simulink model "cruise_control_fechada"  (R2021b)
settings: Solver=FixedStepAuto  StartTime=0.0  StopTime=100.0  FixedStep=1e-3  RelTol=1e-3
values from neighbouring files (symbols this model uses):
  b = b_car + delta_b    [closedDrag.m]    (also in identificarCruiseControl.m = f/v_inf; openDrag.m)
  bc = b    [closedDistur.m]    (also in closedDrag.m = b_car; closedFf.m = 0; closedU.m; closedVelRef.m)
  d = 300    [closedDistur.m]    (also in closedDrag.m = 0; closedFf.m = 0; closedU.m = 0; closedVelRef.m = 0)
  Kp = m/tau - b    [closedDistur.m]    (also in closedDrag.m = m/tau - b_car; closedFf.m; closedU.m; closedVelRef.m)
  m = tau*b    [identificarCruiseControl.m]    (also in openMass.m = m_car + m_pass)
  vr = 10    [closedDistur.m]    (also in closedDrag.m; closedFf.m; closedU.m; closedVelRef.m = 30)
settings Model: Creator=mmaximo  LastModifiedBy=Eric
settings SolverCC: AlgebraicLoopSolver=TrustRegion
settings DebuggingCC: SFMachineParentedDataDiag=warning

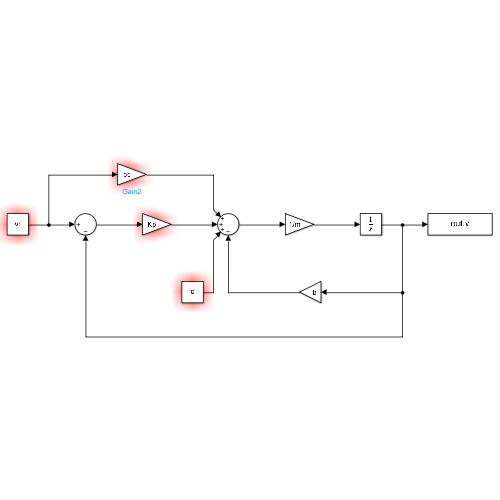
[thumbnail: Simulink's stored preview of the top-level diagram]
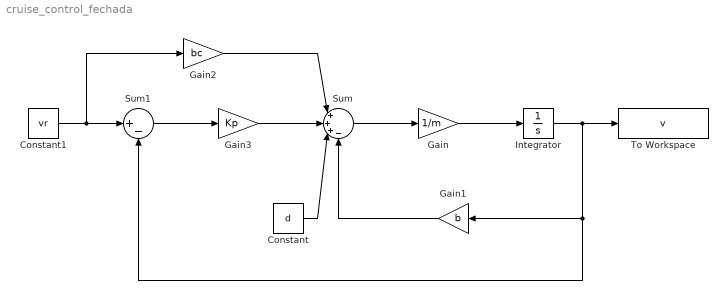
== system cruise_control_fechada ==
  Constant : Constant  Value=d
  Constant1 : Constant  Value=vr
  Gain : Gain  Gain=1/m
  Gain1 : Gain  Gain=b
  Gain2 : Gain  Gain=bc
  Gain3 : Gain  Gain=Kp
  Integrator : Integrator
  Sum : Sum  Inputs=|+++-
  Sum1 : Sum  Inputs=|+-
  To Workspace : ToWorkspace  VariableName=v  SaveFormat=Structure With Time  SampleTime=-1
  wires:
  Constant1/1 -> Gain2/1, Sum1/1
  Gain2/1 -> Sum/1
  Sum1/1 -> Gain3/1
  Gain3/1 -> Sum/2
  Constant/1 -> Sum/3
  Gain1/1 -> Sum/4
  Integrator/1 -> Sum1/2, Gain1/1, To Workspace/1
  Sum/1 -> Gain/1
  Gain/1 -> Integrator/1
